simulink model "impedanceController"  (R2018b)
settings: Solver=VariableStepAuto  StartTime=0.0  StopTime=25  FixedStep=0.1  RelTol=1e-3
libraries: simulink x1
settings Model: Creator=Srikar  LastModifiedBy=holyCow
settings SFSimCC: SimUseLocalCustomCode=off
settings RTWCC: RTWUseLocalCustomCode=off

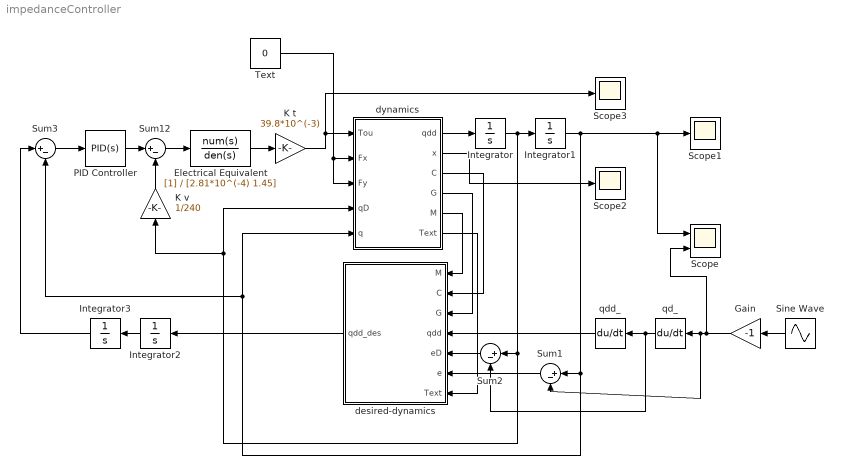
== system impedanceController ==
  Electrical Equivalent : TransferFcn  Denominator=[2.81*10^(-4) 1.45]
  Gain : Gain  Gain=-1
  Integrator{,1..3} (4 alike) : Integrator
  K t : Gain  Gain=39.8*10^(-3)
  K v : Gain  Gain=1/240
  PID Controller : simulink/Continuous/PID Controller  Controller=PID  Form=Parallel  TimeDomain=Continuous-time  SampleTime=-1  IntegratorMethod=Forward Euler  FilterMethod=Forward Euler  ControllerParametersSource=internal  P=1  I=0  D=0  UseFilter=on  N=100  TunerSelectOption=Transfer Function Based (PID Tuner App)  InitialConditionSource=internal  InitialConditionForIntegrator=0  InitialConditionForFilter=0  DifferentiatorICPrevScaledInput=0  ExternalReset=none  TrackingMode=off  Kt=1  LimitOutput=off  UpperSaturationLimit=inf  LowerSaturationLimit=-inf  LinearizeAsGain=on  AntiWindupMode=none  Kb=1  POutMin=[]  POutMax=[]  IOutMin=[]  IOutMax=[]  DOutMin=[]  DOutMax=[]  NOutMin=[]  NOutMax=[]  SumOutMin=[]  SumOutMax=[]  SaturationOutMin=[]  SaturationOutMax=[]  PParamMin=[]  PParamMax=[]  IParamMin=[]  IParamMax=[]  DParamMin=[]  DParamMax=[]  NParamMin=[]  NParamMax=[]  KbParamMin=[]  KbParamMax=[]  KtParamMin=[]  KtParamMax=[]  KbOutMin=[]  KbOutMax=[]  KtOutMin=[]  KtOutMax=[]  IntegratorOutMin=[]  IntegratorOutMax=[]  FilterOutMin=[]  FilterOutMax=[]  SumI1OutMin=[]  SumI1OutMax=[]  SumI2OutMin=[]  SumI2OutMax=[]  SumI3OutMin=[]  SumI3OutMax=[]  SumI4OutMin=[]  SumI4OutMax=[]  SumDOutMin=[]  SumDOutMax=[]  DifferentiatorOutMin=[]  DifferentiatorOutMax=[]  FilterDiffOutCoefMin=[]  FilterDiffOutCoefMax=[]  ReciprocalOutMin=[]  ReciprocalOutMax=[]  SumDenOutMin=[]  SumDenOutMax=[]  SumNumOutMin=[]  SumNumOutMax=[]  DivideOutMin=[]  DivideOutMax=[]  IntegratorContinuousStateAttributes=''  IntegratorStateMustResolveToSignalObject=off  IntegratorRTWStateStorageClass=Auto  FilterContinuousStateAttributes=''  FilterStateMustResolveToSignalObject=off  FilterRTWStateStorageClass=Auto  ParallelPVariant=InternalParameters  IdealPVariant=Disabled  IVariant=InternalParameters  DVariant=InternalParameters  IntegratorVariant=Continuous  SatVariant=Disabled  AWVariant=Passthrough  PCopyVariant=Disabled  TRVariant=Disabled  FdbkBlocksVariant=Forward  IdealPFdbkVariant=Disabled  SatFdbkVariant=Disabled  DerivativeFilterVariant=ContFilter  NVariant=InternalParameters  NCopyVariant=Disabled  FilterICVariant=InternalICsFilter  IntegratorICVariant=InternalICs  ExternalResetVariant=Disabled  TRSumVariant=Passthrough  SumFdbkVariant=Disabled  SumVariant=Sum_PID
  Scope : Scope  NumInputPorts=2
  Scope1 : Scope
  Scope2 : Scope
  Scope3 : Scope
  Sine Wave : Sin  Amplitude=0.5*pi  SampleTime=0
  Sum{1..3,12} (4 alike) : Sum  Inputs=|+-
  Text : Constant  Value=0
  desired-dynamics : MATLAB Function  TreatAsAtomicUnit=on
  dynamics : MATLAB Function  TreatAsAtomicUnit=on
  "qd_ " : Derivative
  qdd_ : Derivative
  wires:
  PID Controller/1 -> Sum12/1
  K t/1 -> Scope3/1, dynamics/1(Tou)
  Integrator1/1 -> Scope/1, Scope1/1, Sum3/2, dynamics/5(q), Sum1/1
  Text/1 -> dynamics/3(Fy), dynamics/2(Fx)
  dynamics/1(qdd) -> Integrator/1
  Electrical Equivalent/1 -> K t/1
  Sum3/1 -> PID Controller/1
  Integrator/1 -> K v/1, dynamics/4(qD), Sum2/1, Integrator1/1
  Sum12/1 -> Electrical Equivalent/1
  K v/1 -> Sum12/2
  dynamics/2(x) -> Scope2/1
  "qd_ "/1 -> Sum2/2, qdd_/1
  Sine Wave/1 -> Gain/1
  qdd_/1 -> desired-dynamics/4(qdd)
  Sum1/1 -> desired-dynamics/6(e)
  Sum2/1 -> desired-dynamics/5(eD)
  desired-dynamics/1(qdd_des) -> Integrator2/1
  dynamics/3(C) -> desired-dynamics/2(C)
  dynamics/4(G) -> desired-dynamics/3(G)
  dynamics/5(M) -> desired-dynamics/1(M)
  dynamics/6(Text) -> desired-dynamics/7(Text)
  Integrator2/1 -> Integrator3/1
  Integrator3/1 -> Sum3/1
  Gain/1 -> Scope/2, Sum1/2, "qd_ "/1

== matlab function impedanceController/desired-dynamics ==
  data: M input; C input; G input; qdd input; eD input; e input; Text input; qdd_des output
function qdd_des = fcn(M, C, G, qdd, eD, e, Text)
l = 0.265;
m = 0.170;
a = 0.110;
b = 0.090;

%params;
Km = 1;
Kb = 1;
Kk = 1;

g = 9.81;

m1 = 2.5;
m2 = 0.2;
mf = 0.075;

% measure of radius
rr = 0.110/2;
rf = 0.075/2;

delta = rr - rf;

% l*sin(q2) + delta = m*sin(q1 - q2)
ta = (l/m + cos(e))^2 + (sin(e))^2;
tb = -2*(delta/m)*sin(e);
tc = (delta/m)^2 - (l/m + cos(e))^2;

q2 = acos((-tb + sqrt(tb^2 - 4*ta*tc))/(2*ta));
k = 1/(1 + ((l*cos(q2))/(m*cos(e - q2))));
%q2D = k * q1D;

x = sqrt(l^2 + m^2 - delta^2 + 2*l*m*cos(e));
c = ((-l*m*sin(e))/x);
%xD = c * q1D;

s = (l*k*m*sin(q2)*cos(e - q2) - l*m*cos(q2)*sin(e - q2)*(1 - k))/((l*cos(q2) + m*cos(e - q2))^2);
u = (l*m*(c*sin(e) - x*cos(e)))/(x^2);

%kD = s * q1D;
%cD = u * q1D;

%xa = a*cos(q2);
%xaD = -a*sin(q2)*q2D;

%ya = rr + a*sin(q2);
%yaD = a*cos(q2)*q2D;

%xb = x - b*cos(q - q2);
%xbD = xD + b*sin(q1 - q2)*(q1D - q2D);

%yb = rf + b*sin(q1 - q2);
%ybD = b*cos(q1 - q2)*(q1D - q2D);

%K = 0.5*m1*(xaD^2 + yaD^2) + 0.5*m2*(xbD^2 + ybD^2) + 0.75*mf*xD^2;
%P = mr*g*rr + mf*g*rf + m1*g*ya + m2*g*yb;

Md = m1*(a^2)*(k^2) + (m2 + 1.5*mf)*(c^2) + m2*(b^2)*((1-k)^2) + 2*m2*b*sin(e - q2)*c*(1-k);

ctemp = cos(e - q2)*c*((1-k)^2) + sin(e - q2)*u*(1-k) - sin(e - q2)*c*s;
Bd = (m1*(a^2)*k*s + (m2 + 1.5*mf)*c*u - m2*(b^2)*s*(1-k) + m2*b*ctemp) * (eD^2);

Kd = m1*g*a*cos(q2)*k + m2*g*b*cos(e - q2)*(1 - k);

%N2 = (m1*g*xa + m2*g*xb)/(x);
%N1 = (((m1+m2)*x - m1*xa - m2*xb)*g)/(x);
%T_ext = Text + N1*l*cos(q2) - N2*m*cos(q1 - q2);
qdd_des = qdd - (Text + Kb*Bd + Kk*Kd)/(Km*Md);

== matlab function impedanceController/dynamics ==
  data: Tou input; Fx input; Fy input; qD input; qdd output; q input; x output; C output; G output; M output; Text output
function [qdd, x, C, G, M, Text]= fcn(Tou, Fx, Fy, qD, q)
l = 0.265;
m = 0.170;
a = 0.110;
b = 0.090;

g = 9.81;

m1 = 2.5;
m2 = 0.2;
mr = 0.1;
mf = 0.075;

% measure of radius
rr = 0.110/2;
rf = 0.075/2;

delta = rr - rf;

% l*sin(q2) + delta = m*sin(q1 - q2)
ta = (l/m + cos(q))^2 + (sin(q))^2;
tb = -2*(delta/m)*sin(q);
tc = (delta/m)^2 - (l/m + cos(q))^2;

q2 = acos((-tb + sqrt(tb^2 - 4*ta*tc))/(2*ta));
k = 1/(1 + ((l*cos(q2))/(m*cos(q - q2))));
%q2D = k * q1D;

x = sqrt(l^2 + m^2 - delta^2 + 2*l*m*cos(q));
c = ((-l*m*sin(q))/x);
%xD = c * q1D;

s = (l*k*m*sin(q2)*cos(q - q2) - l*m*cos(q2)*sin(q - q2)*(1 - k))/((l*cos(q2) + m*cos(q - q2))^2);
u = (l*m*(c*sin(q) - x*cos(q)))/(x^2);

%kD = s * q1D;
%cD = u * q1D;

%xa = a*cos(q2);
%xaD = -a*sin(q2)*q2D;

%ya = rr + a*sin(q2);
%yaD = a*cos(q2)*q2D;

%xb = x - b*cos(q - q2);
%xbD = xD + b*sin(q1 - q2)*(q1D - q2D);

%yb = rf + b*sin(q1 - q2);
%ybD = b*cos(q1 - q2)*(q1D - q2D);

%K = 0.5*m1*(xaD^2 + yaD^2) + 0.5*m2*(xbD^2 + ybD^2) + 0.75*mf*xD^2;
%P = mr*g*rr + mf*g*rf + m1*g*ya + m2*g*yb;

M = m1*(a^2)*(k^2) + (m2 + 1.5*mf)*(c^2) + m2*(b^2)*((1-k)^2) + 2*m2*b*sin(q - q2)*c*(1-k);

ctemp = cos(q - q2)*c*((1-k)^2) + sin(q - q2)*u*(1-k) - sin(q - q2)*c*s;
C = (m1*(a^2)*k*s + (m2 + 1.5*mf)*c*u - m2*(b^2)*s*(1-k) + m2*b*ctemp) * (qD^2);

G = m1*g*a*cos(q2)*k + m2*g*b*cos(q - q2)*(1 - k);

%N2 = (m1*g*xa + m2*g*xb)/(x);
%N1 = (((m1+m2)*x - m1*xa - m2*xb)*g)/(x);
%T_ext = Text + N1*l*cos(q2) - N2*m*cos(q1 - q2);
Text = Fx*l*sin(q - q2) - Fy*m*cos(q - q2);
qdd = (Tou - Text - C - G)/M;
